simulink model "bounce_converge"  (R2023b)
settings: Solver=VariableStepAuto  StartTime=0.0  StopTime=10.0  RelTol=1e-3
libraries: simulink x1
settings Model: Creator=awcm9  LastModifiedBy=awcm9

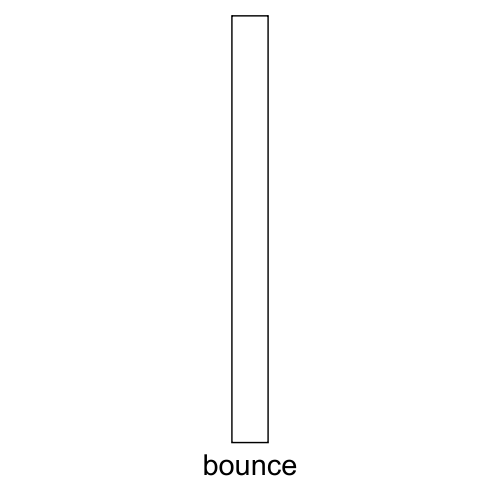
[thumbnail: Simulink's stored preview of the top-level diagram]
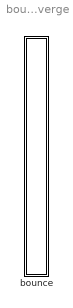
== system bounce_converge ==
  bounce : Subsystem

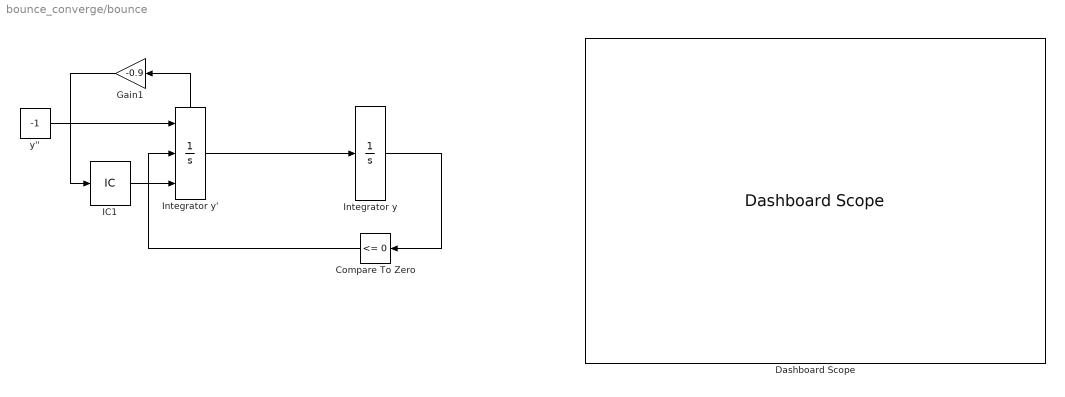
== system bounce_converge/bounce ==
  Compare To Zero : simulink/Logic and Bit Operations/Compare To Zero  relop=<=  OutDataTypeStr=boolean
  Dashboard Scope : DashboardScope  ShowInitialText=off  TimeSpan=10  Ymin=-.25  Ymax=1.25  ScaleAtStop=off  UpdateMode=Scroll
  Gain1 : Gain  Gain=-0.9
  IC1 : InitialCondition
  Integrator y : Integrator  InitialCondition=0.5  LimitOutput=on  UpperSaturationLimit=10  LowerSaturationLimit=0  ZeroCross=off
  Integrator y' : Integrator  ExternalReset=rising  InitialConditionSource=external  ShowStatePort=on  ZeroCross=off
  y'' : Constant  Value=-1
  wires:
  Integrator y'/1 -> Integrator y/1
  y''/1 -> Integrator y'/1
  Gain1/1 -> IC1/1
  IC1/1 -> Integrator y'/3
  Integrator y'/State -> Gain1/1
  Compare To Zero/1 -> Integrator y'/2
  Integrator y/1 -> Compare To Zero/1
